simulink library "neuronpoolib"  (Simulink 7.6)
settings: Solver=ode45  StartTime=0.0  StopTime=10.0  RelTol=1e-3
values from neighbouring files (symbols this model uses):
  amp = 1    [excneuroninit.m]
  ampe = 0.5    [excneuroninit.m]
  h = -0.5    [excneuroninit.m]
  maxcon = 10    [excneuroninit.m]
  neurodist = 1    [excneuroninit.m]
  sigslope = 3    [excneuroninit.m]
  tau_u = 0.05    [excneuroninit.m]
  tau_v = 0.1    [excneuroninit.m]
libraries: simulink x20
settings Model: Creator=root  LastModifiedBy=root

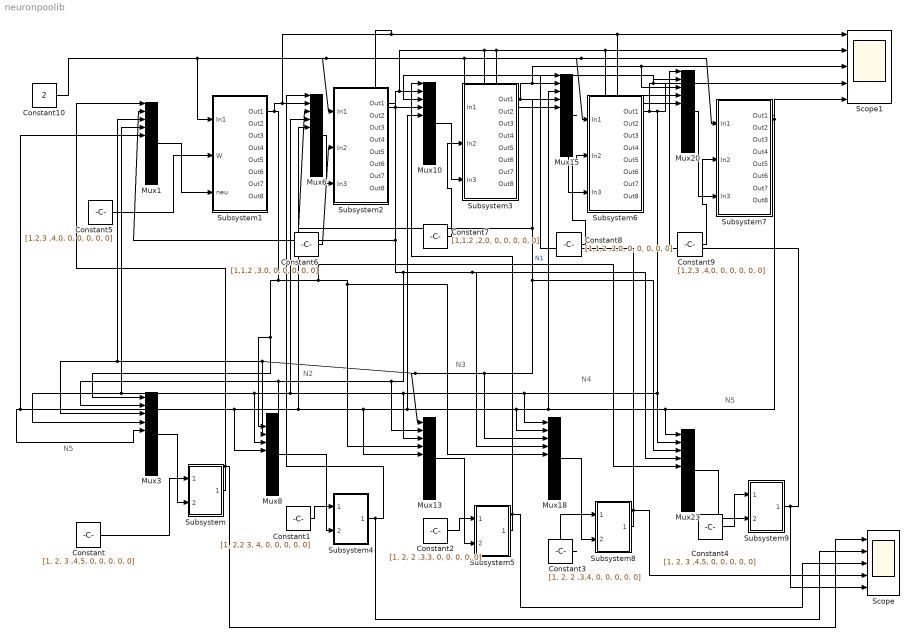
== system neuronpoolib ==
  note: N5
  note: N5
  note: N4
  note: N3
  note: N2
  Constant : Constant  Value=[1, 2, 3 ,4,5, 0, 0, 0, 0, 0]
  Constant1 : Constant  Value=[1, 2,2 3, 4, 0, 0, 0, 0, 0]
  Constant10 : Constant  Value=2
  Constant2 : Constant  Value=[1, 2, 2 ,3,3, 0, 0, 0, 0, 0]
  Constant3 : Constant  Value=[1, 2, 2 ,3,4, 0, 0, 0, 0, 0]
  Constant4 : Constant  Value=[1, 2, 3 ,4,5, 0, 0, 0, 0, 0]
  Constant5 : Constant  Value=[1,2,3 ,4,0, 0, 0, 0, 0, 0]
  Constant6 : Constant  Value=[1,1,2 ,3,0, 0, 0, 0, 0, 0]
  Constant7 : Constant  Value=[1,1,2 ,2,0, 0, 0, 0, 0, 0]
  Constant8 : Constant  Value=[1,1,2 ,3,0, 0, 0, 0, 0, 0]
  Constant9 : Constant  Value=[1,2,3 ,4,0, 0, 0, 0, 0, 0]
  Mux{1,6,10,15,20} (5 alike) : Mux  Inputs=11
  Mux{3,8,13,18,23} (5 alike) : Mux  Inputs=10
  Scope : Scope  NumInputPorts=5
      settings: YMin=-5~-5~-5~-5~-5  YMax=5~5~5~5~5
  Scope1 : Scope  NumInputPorts=5
      settings: YMin=-5~-5~-5~-5~-5  YMax=5~5~5~5~5
  Subsystem : Subsystem
  Subsystem1 : Subsystem
  Subsystem2 : Subsystem
  Subsystem3 : Subsystem
  Subsystem4 : Subsystem
  Subsystem5 : Subsystem
  Subsystem6 : Subsystem
  Subsystem7 : Subsystem
  Subsystem8 : Subsystem
  Subsystem9 : Subsystem
  wires:
  Subsystem1/1(Out1) -> Mux6/2, Mux10/4, Scope1/1, Mux20/5, Mux3/1, Mux8/2, Mux13/4, Mux18/5, Mux23/5  "N1"
  Subsystem2/1(Out1) -> Mux10/2, Mux15/4, Scope1/2, Mux20/4, Mux15/5, Mux3/2, Mux8/1, Mux13/2, Mux18/4, Mux23/4, Mux1/2
  Subsystem3/1(Out1) -> Mux8/3, Mux3/3, Mux1/3, Mux13/1, Mux18/3, Mux23/3, Mux6/3, Mux15/2, Scope1/3, Mux20/3
  Subsystem6/1(Out1) -> Mux18/1, Mux13/3, Mux8/4, Mux3/4, Mux1/4, Mux6/4, Mux23/2, Mux10/3, Mux20/2, Scope1/4
  Subsystem7/1(Out1) -> Mux23/1, Mux18/2, Mux13/5, Mux8/5, Mux3/5, Mux1/5, Mux6/5, Mux10/5, Mux15/3, Scope1/5
  Mux3/1 -> Subsystem/2(port2)
  Mux8/1 -> Subsystem4/2(port2)
  Mux13/1 -> Subsystem5/2(port2)
  Mux18/1 -> Subsystem8/2(port2)
  Mux23/1 -> Subsystem9/2(port2)
  Constant10/1 -> Subsystem2/1(In1), Subsystem7/1(In1), Subsystem6/1(In1), Subsystem3/1(In1), Subsystem1/1(In1)
  Subsystem/1(Out2) -> Mux1/1, Scope/1
  Subsystem4/1(Out2) -> Mux6/1, Scope/2
  Subsystem5/1(Out2) -> Mux10/1, Scope/3
  Subsystem8/1(Out2) -> Mux15/1, Scope/4
  Subsystem9/1(Out2) -> Mux20/1, Scope/5
  Mux1/1 -> Subsystem1/3(neu)
  Mux6/1 -> Subsystem2/3(In3)
  Mux10/1 -> Subsystem3/3(In3)
  Mux15/1 -> Subsystem6/3(In3)
  Mux20/1 -> Subsystem7/3(In3)
  Constant/1 -> Subsystem/1(port1)
  Constant1/1 -> Subsystem4/1(port1)
  ? -> ?
  Constant2/1 -> Subsystem5/1(port1)
  Constant3/1 -> Subsystem8/1(port1)
  Constant4/1 -> Subsystem9/1(port1)
  Constant5/1 -> Subsystem1/2(W)
  Constant6/1 -> Subsystem2/2(In2)
  Constant7/1 -> Subsystem3/2(In2)
  Constant8/1 -> Subsystem6/2(In2)
  Constant9/1 -> Subsystem7/2(In2)

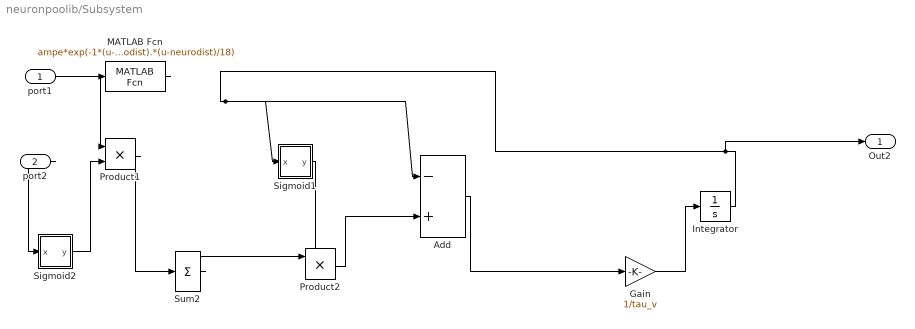
== system neuronpoolib/Subsystem ==
  port1 : Inport
  port2 : Inport  Port=2
  Add : Sum  Inputs=-+
  Gain : Gain  Gain=1/tau_v
  Integrator : Integrator  InitialCondition=1
  MATLAB Fcn : MATLABFcn  MATLABFcn=ampe*exp(-1*(u-neurodist).*(u-neurodist)/18)  OutputDimensions=maxcon
  Product1 : Product  RndMeth=Zero
  Product2 : Product  RndMeth=Zero
  Sigmoid1 : Subsystem  TreatAsAtomicUnit=on  mask{slope=sigslope, offset=0.5}
      mask help: Created by Han, Cheol
      mask Display: plot([10 15 20 25 30 35 40 45 50], [0 0.01 0.1 0.2 0.5 0.8 0.9 0.99 1])
  Sigmoid2 : Subsystem  TreatAsAtomicUnit=on  mask{slope=sigslope, offset=0.5}
      mask help: Created by Han, Cheol
      mask Display: plot([10 15 20 25 30 35 40 45 50], [0 0.01 0.1 0.2 0.5 0.8 0.9 0.99 1])
  Sum2 : Sum  Inputs=+  SaturateOnIntegerOverflow=on
  Out2 : Outport
  wires:
  Add/1 -> Gain/1
  Gain/1 -> Integrator/1
  Integrator/1 -> Add/1, Sigmoid1/1(x), Out2/1
  MATLAB Fcn/1 -> Product1/1
  Sigmoid2/1(y) -> Product1/2
  Product1/1 -> Sum2/1
  Sum2/1 -> Product2/1
  Sigmoid1/1(y) -> Product2/2
  port1/1 -> MATLAB Fcn/1
  port2/1 -> Sigmoid2/1(x)
  Product2/1 -> Add/2

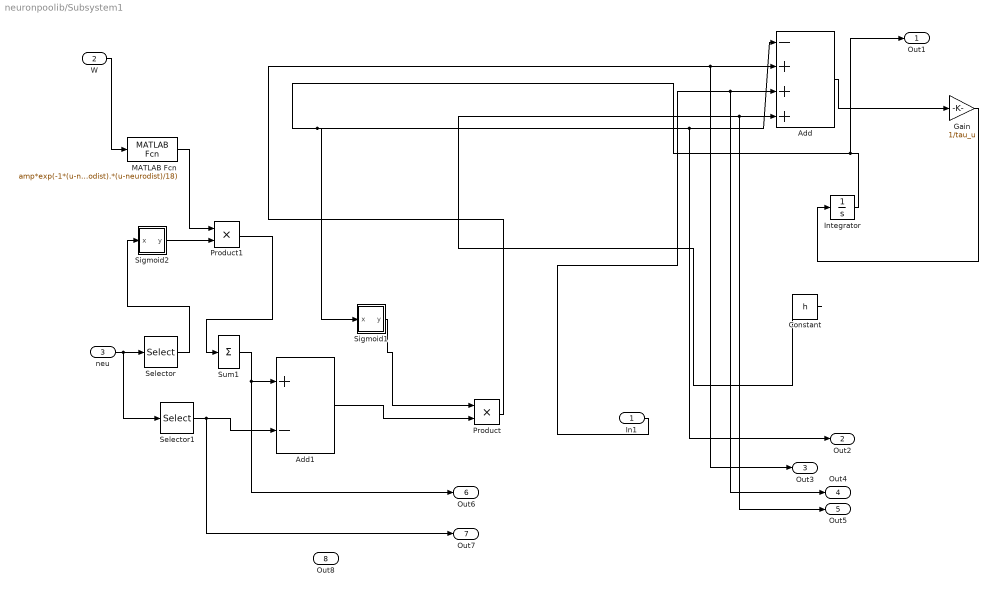
== system neuronpoolib/Subsystem1 ==
  In1 : Inport
  W : Inport  Port=2
  neu : Inport  Port=3
  Add : Sum  Inputs=-+++
  Add1 : Sum  Inputs=+-
  Constant : Constant  Value=h
  Gain : Gain  Gain=1/tau_u
  Integrator : Integrator  InitialCondition=1
  MATLAB Fcn : MATLABFcn  MATLABFcn=amp*exp(-1*(u-neurodist).*(u-neurodist)/18)  OutputDimensions=maxcon
  Product : Product  RndMeth=Zero
  Product1 : Product  RndMeth=Zero
  Selector : Selector  InputPortWidth=maxcon+1  IndexOptions=Starting index (dialog)  Indices=2  OutputSizes=maxcon
  Selector1 : Selector  InputPortWidth=maxcon+1  IndexOptions=Starting index (dialog)  Indices=1  OutputSizes=1
  Sigmoid1 : Subsystem  TreatAsAtomicUnit=on  mask{slope=sigslope, offset=0.5}
      mask help: Created by Han, Cheol
      mask Display: plot([10 15 20 25 30 35 40 45 50], [0 0.01 0.1 0.2 0.5 0.8 0.9 0.99 1])
  Sigmoid2 : Subsystem  TreatAsAtomicUnit=on  mask{slope=sigslope, offset=0.5}
      mask help: Created by Han, Cheol
      mask Display: plot([10 15 20 25 30 35 40 45 50], [0 0.01 0.1 0.2 0.5 0.8 0.9 0.99 1])
  Sum1 : Sum  Inputs=+  SaturateOnIntegerOverflow=on
  Out1 : Outport
  Out2 : Outport  Port=2
  Out3 : Outport  Port=3
  Out4 : Outport  Port=4
  Out5 : Outport  Port=5
  Out6 : Outport  Port=6
  Out7 : Outport  Port=7
  Out8 : Outport  Port=8
  wires:
  Add/1 -> Gain/1
  Gain/1 -> Integrator/1
  Integrator/1 -> Sigmoid1/1(x), Add/1, Out2/1, Out1/1
  Sigmoid1/1(y) -> Product/1
  Product/1 -> Add/2, Out3/1
  In1/1 -> Add/3, Out4/1
  Constant/1 -> Add/4, Out5/1
  neu/1 -> Selector/1, Selector1/1
  Product1/1 -> Sum1/1
  Selector/1 -> Sigmoid2/1(x)
  W/1 -> MATLAB Fcn/1
  MATLAB Fcn/1 -> Product1/1
  Sum1/1 -> Add1/1, Out6/1
  Selector1/1 -> Add1/2, Out7/1
  Sigmoid2/1(y) -> Product1/2
  Add1/1 -> Product/2

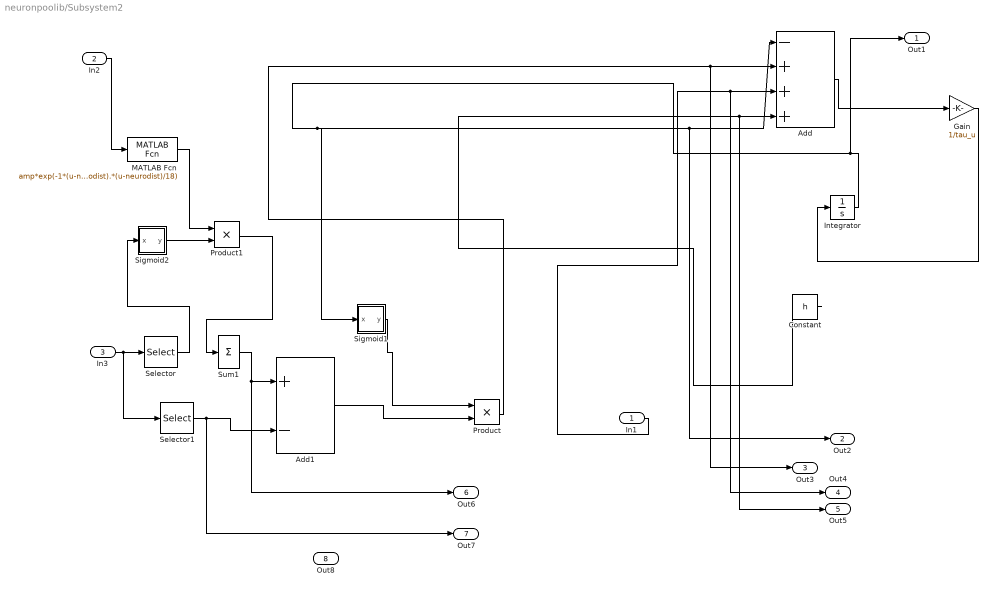
== system neuronpoolib/Subsystem2 ==
  In1 : Inport
  In2 : Inport  Port=2
  In3 : Inport  Port=3
  Add : Sum  Inputs=-+++
  Add1 : Sum  Inputs=+-
  Constant : Constant  Value=h
  Gain : Gain  Gain=1/tau_u
  Integrator : Integrator  InitialCondition=1
  MATLAB Fcn : MATLABFcn  MATLABFcn=amp*exp(-1*(u-neurodist).*(u-neurodist)/18)  OutputDimensions=maxcon
  Product : Product  RndMeth=Zero
  Product1 : Product  RndMeth=Zero
  Selector : Selector  InputPortWidth=maxcon+1  IndexOptions=Starting index (dialog)  Indices=2  OutputSizes=maxcon
  Selector1 : Selector  InputPortWidth=maxcon+1  IndexOptions=Starting index (dialog)  Indices=1  OutputSizes=1
  Sigmoid1 : Subsystem  TreatAsAtomicUnit=on  mask{slope=sigslope, offset=0.5}
      mask help: Created by Han, Cheol
      mask Display: plot([10 15 20 25 30 35 40 45 50], [0 0.01 0.1 0.2 0.5 0.8 0.9 0.99 1])
  Sigmoid2 : Subsystem  TreatAsAtomicUnit=on  mask{slope=sigslope, offset=0.5}
      mask help: Created by Han, Cheol
      mask Display: plot([10 15 20 25 30 35 40 45 50], [0 0.01 0.1 0.2 0.5 0.8 0.9 0.99 1])
  Sum1 : Sum  Inputs=+  SaturateOnIntegerOverflow=on
  Out1 : Outport
  Out2 : Outport  Port=2
  Out3 : Outport  Port=3
  Out4 : Outport  Port=4
  Out5 : Outport  Port=5
  Out6 : Outport  Port=6
  Out7 : Outport  Port=7
  Out8 : Outport  Port=8
  wires:
  Add/1 -> Gain/1
  Gain/1 -> Integrator/1
  Integrator/1 -> Sigmoid1/1(x), Add/1, Out2/1, Out1/1
  Sigmoid1/1(y) -> Product/1
  Product/1 -> Add/2, Out3/1
  In1/1 -> Add/3, Out4/1
  Constant/1 -> Add/4, Out5/1
  In3/1 -> Selector/1, Selector1/1
  Product1/1 -> Sum1/1
  Selector/1 -> Sigmoid2/1(x)
  In2/1 -> MATLAB Fcn/1
  MATLAB Fcn/1 -> Product1/1
  Sum1/1 -> Add1/1, Out6/1
  Selector1/1 -> Add1/2, Out7/1
  Sigmoid2/1(y) -> Product1/2
  Add1/1 -> Product/2

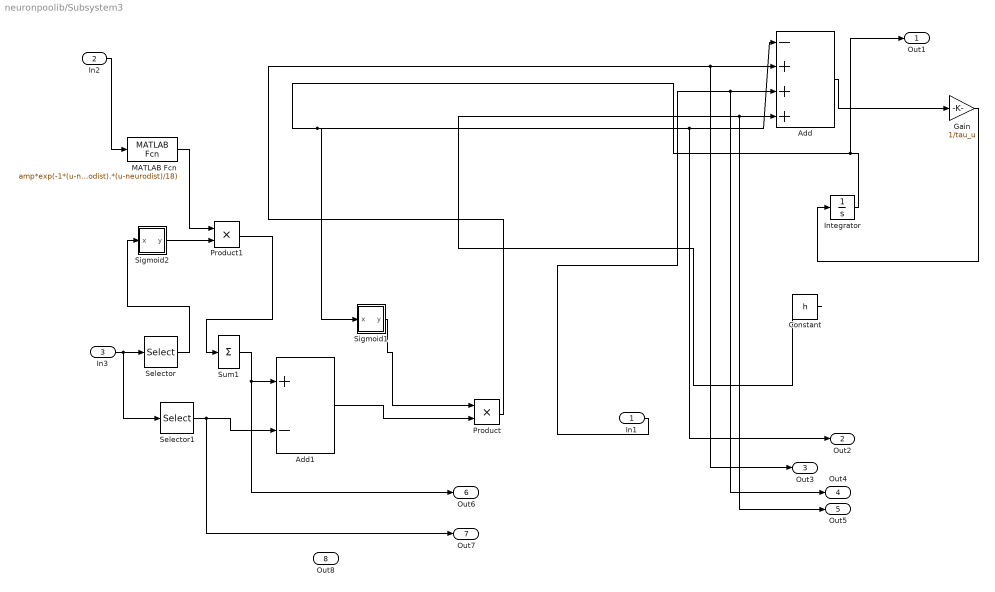
== system neuronpoolib/Subsystem3 ==
  In1 : Inport
  In2 : Inport  Port=2
  In3 : Inport  Port=3
  Add : Sum  Inputs=-+++
  Add1 : Sum  Inputs=+-
  Constant : Constant  Value=h
  Gain : Gain  Gain=1/tau_u
  Integrator : Integrator  InitialCondition=1
  MATLAB Fcn : MATLABFcn  MATLABFcn=amp*exp(-1*(u-neurodist).*(u-neurodist)/18)  OutputDimensions=maxcon
  Product : Product  RndMeth=Zero
  Product1 : Product  RndMeth=Zero
  Selector : Selector  InputPortWidth=maxcon+1  IndexOptions=Starting index (dialog)  Indices=2  OutputSizes=maxcon
  Selector1 : Selector  InputPortWidth=maxcon+1  IndexOptions=Starting index (dialog)  Indices=1  OutputSizes=1
  Sigmoid1 : Subsystem  TreatAsAtomicUnit=on  mask{slope=sigslope, offset=0.5}
      mask help: Created by Han, Cheol
      mask Display: plot([10 15 20 25 30 35 40 45 50], [0 0.01 0.1 0.2 0.5 0.8 0.9 0.99 1])
  Sigmoid2 : Subsystem  TreatAsAtomicUnit=on  mask{slope=sigslope, offset=0.5}
      mask help: Created by Han, Cheol
      mask Display: plot([10 15 20 25 30 35 40 45 50], [0 0.01 0.1 0.2 0.5 0.8 0.9 0.99 1])
  Sum1 : Sum  Inputs=+  SaturateOnIntegerOverflow=on
  Out1 : Outport
  Out2 : Outport  Port=2
  Out3 : Outport  Port=3
  Out4 : Outport  Port=4
  Out5 : Outport  Port=5
  Out6 : Outport  Port=6
  Out7 : Outport  Port=7
  Out8 : Outport  Port=8
  wires:
  Add/1 -> Gain/1
  Gain/1 -> Integrator/1
  Integrator/1 -> Sigmoid1/1(x), Add/1, Out2/1, Out1/1
  Sigmoid1/1(y) -> Product/1
  Product/1 -> Add/2, Out3/1
  In1/1 -> Add/3, Out4/1
  Constant/1 -> Add/4, Out5/1
  In3/1 -> Selector/1, Selector1/1
  Product1/1 -> Sum1/1
  Selector/1 -> Sigmoid2/1(x)
  In2/1 -> MATLAB Fcn/1
  MATLAB Fcn/1 -> Product1/1
  Sum1/1 -> Add1/1, Out6/1
  Selector1/1 -> Add1/2, Out7/1
  Sigmoid2/1(y) -> Product1/2
  Add1/1 -> Product/2

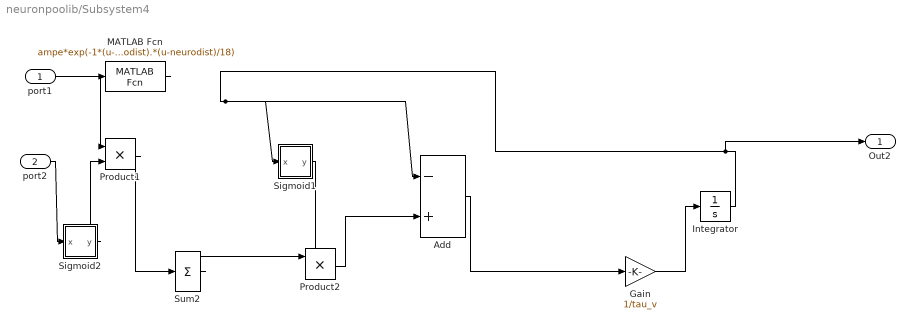
== system neuronpoolib/Subsystem4 ==
  port1 : Inport
  port2 : Inport  Port=2
  Add : Sum  Inputs=-+
  Gain : Gain  Gain=1/tau_v
  Integrator : Integrator  InitialCondition=1
  MATLAB Fcn : MATLABFcn  MATLABFcn=ampe*exp(-1*(u-neurodist).*(u-neurodist)/18)  OutputDimensions=maxcon
  Product1 : Product  RndMeth=Zero
  Product2 : Product  RndMeth=Zero
  Sigmoid1 : Subsystem  TreatAsAtomicUnit=on  mask{slope=sigslope, offset=0.5}
      mask help: Created by Han, Cheol
      mask Display: plot([10 15 20 25 30 35 40 45 50], [0 0.01 0.1 0.2 0.5 0.8 0.9 0.99 1])
  Sigmoid2 : Subsystem  TreatAsAtomicUnit=on  mask{slope=sigslope, offset=0.5}
      mask help: Created by Han, Cheol
      mask Display: plot([10 15 20 25 30 35 40 45 50], [0 0.01 0.1 0.2 0.5 0.8 0.9 0.99 1])
  Sum2 : Sum  Inputs=+  SaturateOnIntegerOverflow=on
  Out2 : Outport
  wires:
  Add/1 -> Gain/1
  Gain/1 -> Integrator/1
  Integrator/1 -> Add/1, Sigmoid1/1(x), Out2/1
  MATLAB Fcn/1 -> Product1/1
  Sigmoid2/1(y) -> Product1/2
  Product1/1 -> Sum2/1
  Sum2/1 -> Product2/1
  Sigmoid1/1(y) -> Product2/2
  port1/1 -> MATLAB Fcn/1
  port2/1 -> Sigmoid2/1(x)
  Product2/1 -> Add/2

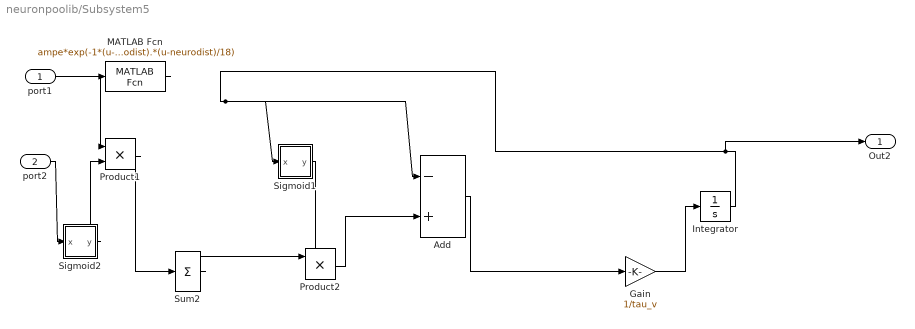
== system neuronpoolib/Subsystem5 ==
  port1 : Inport
  port2 : Inport  Port=2
  Add : Sum  Inputs=-+
  Gain : Gain  Gain=1/tau_v
  Integrator : Integrator  InitialCondition=1
  MATLAB Fcn : MATLABFcn  MATLABFcn=ampe*exp(-1*(u-neurodist).*(u-neurodist)/18)  OutputDimensions=maxcon
  Product1 : Product  RndMeth=Zero
  Product2 : Product  RndMeth=Zero
  Sigmoid1 : Subsystem  TreatAsAtomicUnit=on  mask{slope=sigslope, offset=0.5}
      mask help: Created by Han, Cheol
      mask Display: plot([10 15 20 25 30 35 40 45 50], [0 0.01 0.1 0.2 0.5 0.8 0.9 0.99 1])
  Sigmoid2 : Subsystem  TreatAsAtomicUnit=on  mask{slope=sigslope, offset=0.5}
      mask help: Created by Han, Cheol
      mask Display: plot([10 15 20 25 30 35 40 45 50], [0 0.01 0.1 0.2 0.5 0.8 0.9 0.99 1])
  Sum2 : Sum  Inputs=+  SaturateOnIntegerOverflow=on
  Out2 : Outport
  wires:
  Add/1 -> Gain/1
  Gain/1 -> Integrator/1
  Integrator/1 -> Add/1, Sigmoid1/1(x), Out2/1
  MATLAB Fcn/1 -> Product1/1
  Sigmoid2/1(y) -> Product1/2
  Product1/1 -> Sum2/1
  Sum2/1 -> Product2/1
  Sigmoid1/1(y) -> Product2/2
  port1/1 -> MATLAB Fcn/1
  port2/1 -> Sigmoid2/1(x)
  Product2/1 -> Add/2

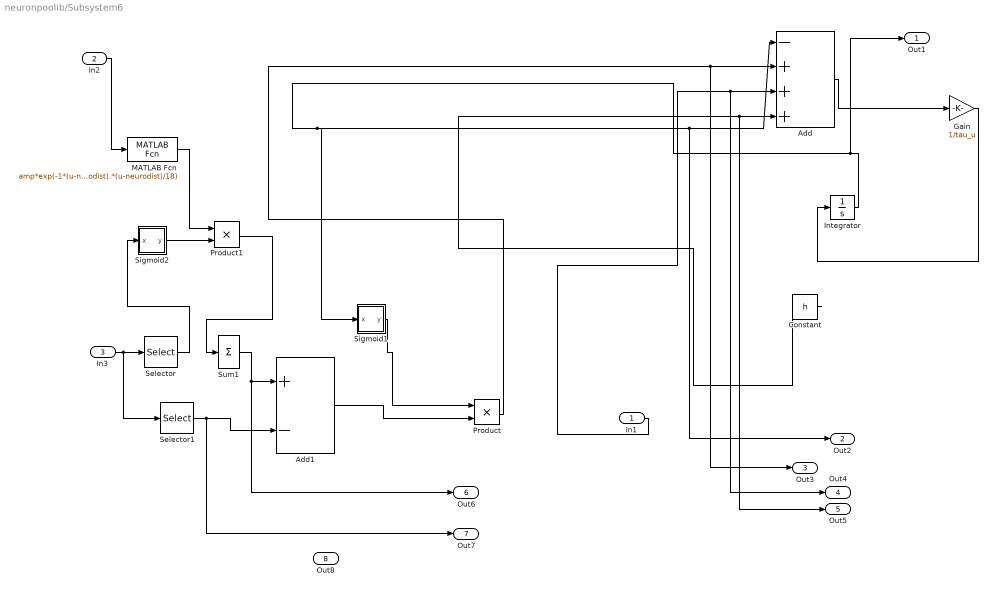
== system neuronpoolib/Subsystem6 ==
  In1 : Inport
  In2 : Inport  Port=2
  In3 : Inport  Port=3
  Add : Sum  Inputs=-+++
  Add1 : Sum  Inputs=+-
  Constant : Constant  Value=h
  Gain : Gain  Gain=1/tau_u
  Integrator : Integrator  InitialCondition=1
  MATLAB Fcn : MATLABFcn  MATLABFcn=amp*exp(-1*(u-neurodist).*(u-neurodist)/18)  OutputDimensions=maxcon
  Product : Product  RndMeth=Zero
  Product1 : Product  RndMeth=Zero
  Selector : Selector  InputPortWidth=maxcon+1  IndexOptions=Starting index (dialog)  Indices=2  OutputSizes=maxcon
  Selector1 : Selector  InputPortWidth=maxcon+1  IndexOptions=Starting index (dialog)  Indices=1  OutputSizes=1
  Sigmoid1 : Subsystem  TreatAsAtomicUnit=on  mask{slope=sigslope, offset=0.5}
      mask help: Created by Han, Cheol
      mask Display: plot([10 15 20 25 30 35 40 45 50], [0 0.01 0.1 0.2 0.5 0.8 0.9 0.99 1])
  Sigmoid2 : Subsystem  TreatAsAtomicUnit=on  mask{slope=sigslope, offset=0.5}
      mask help: Created by Han, Cheol
      mask Display: plot([10 15 20 25 30 35 40 45 50], [0 0.01 0.1 0.2 0.5 0.8 0.9 0.99 1])
  Sum1 : Sum  Inputs=+  SaturateOnIntegerOverflow=on
  Out1 : Outport
  Out2 : Outport  Port=2
  Out3 : Outport  Port=3
  Out4 : Outport  Port=4
  Out5 : Outport  Port=5
  Out6 : Outport  Port=6
  Out7 : Outport  Port=7
  Out8 : Outport  Port=8
  wires:
  Add/1 -> Gain/1
  Gain/1 -> Integrator/1
  Integrator/1 -> Sigmoid1/1(x), Add/1, Out2/1, Out1/1
  Sigmoid1/1(y) -> Product/1
  Product/1 -> Add/2, Out3/1
  In1/1 -> Add/3, Out4/1
  Constant/1 -> Add/4, Out5/1
  In3/1 -> Selector/1, Selector1/1
  Product1/1 -> Sum1/1
  Selector/1 -> Sigmoid2/1(x)
  In2/1 -> MATLAB Fcn/1
  MATLAB Fcn/1 -> Product1/1
  Sum1/1 -> Add1/1, Out6/1
  Selector1/1 -> Add1/2, Out7/1
  Sigmoid2/1(y) -> Product1/2
  Add1/1 -> Product/2

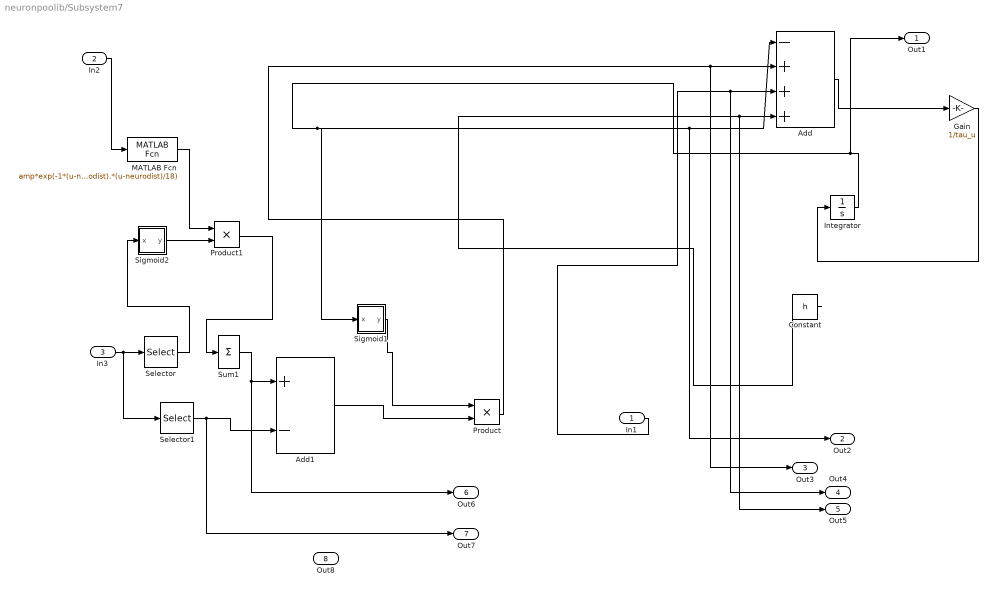
== system neuronpoolib/Subsystem7 ==
  In1 : Inport
  In2 : Inport  Port=2
  In3 : Inport  Port=3
  Add : Sum  Inputs=-+++
  Add1 : Sum  Inputs=+-
  Constant : Constant  Value=h
  Gain : Gain  Gain=1/tau_u
  Integrator : Integrator  InitialCondition=1
  MATLAB Fcn : MATLABFcn  MATLABFcn=amp*exp(-1*(u-neurodist).*(u-neurodist)/18)  OutputDimensions=maxcon
  Product : Product  RndMeth=Zero
  Product1 : Product  RndMeth=Zero
  Selector : Selector  InputPortWidth=maxcon+1  IndexOptions=Starting index (dialog)  Indices=2  OutputSizes=maxcon
  Selector1 : Selector  InputPortWidth=maxcon+1  IndexOptions=Starting index (dialog)  Indices=1  OutputSizes=1
  Sigmoid1 : Subsystem  TreatAsAtomicUnit=on  mask{slope=sigslope, offset=0.5}
      mask help: Created by Han, Cheol
      mask Display: plot([10 15 20 25 30 35 40 45 50], [0 0.01 0.1 0.2 0.5 0.8 0.9 0.99 1])
  Sigmoid2 : Subsystem  TreatAsAtomicUnit=on  mask{slope=sigslope, offset=0.5}
      mask help: Created by Han, Cheol
      mask Display: plot([10 15 20 25 30 35 40 45 50], [0 0.01 0.1 0.2 0.5 0.8 0.9 0.99 1])
  Sum1 : Sum  Inputs=+  SaturateOnIntegerOverflow=on
  Out1 : Outport
  Out2 : Outport  Port=2
  Out3 : Outport  Port=3
  Out4 : Outport  Port=4
  Out5 : Outport  Port=5
  Out6 : Outport  Port=6
  Out7 : Outport  Port=7
  Out8 : Outport  Port=8
  wires:
  Add/1 -> Gain/1
  Gain/1 -> Integrator/1
  Integrator/1 -> Sigmoid1/1(x), Add/1, Out2/1, Out1/1
  Sigmoid1/1(y) -> Product/1
  Product/1 -> Add/2, Out3/1
  In1/1 -> Add/3, Out4/1
  Constant/1 -> Add/4, Out5/1
  In3/1 -> Selector/1, Selector1/1
  Product1/1 -> Sum1/1
  Selector/1 -> Sigmoid2/1(x)
  In2/1 -> MATLAB Fcn/1
  MATLAB Fcn/1 -> Product1/1
  Sum1/1 -> Add1/1, Out6/1
  Selector1/1 -> Add1/2, Out7/1
  Sigmoid2/1(y) -> Product1/2
  Add1/1 -> Product/2

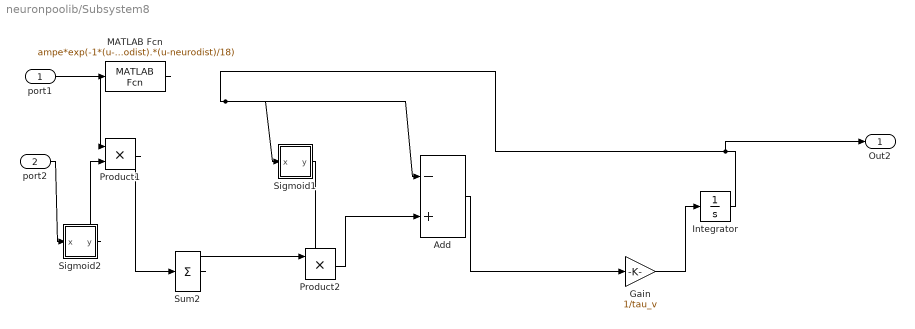
== system neuronpoolib/Subsystem8 ==
  port1 : Inport
  port2 : Inport  Port=2
  Add : Sum  Inputs=-+
  Gain : Gain  Gain=1/tau_v
  Integrator : Integrator  InitialCondition=1
  MATLAB Fcn : MATLABFcn  MATLABFcn=ampe*exp(-1*(u-neurodist).*(u-neurodist)/18)  OutputDimensions=maxcon
  Product1 : Product  RndMeth=Zero
  Product2 : Product  RndMeth=Zero
  Sigmoid1 : Subsystem  TreatAsAtomicUnit=on  mask{slope=sigslope, offset=0.5}
      mask help: Created by Han, Cheol
      mask Display: plot([10 15 20 25 30 35 40 45 50], [0 0.01 0.1 0.2 0.5 0.8 0.9 0.99 1])
  Sigmoid2 : Subsystem  TreatAsAtomicUnit=on  mask{slope=sigslope, offset=0.5}
      mask help: Created by Han, Cheol
      mask Display: plot([10 15 20 25 30 35 40 45 50], [0 0.01 0.1 0.2 0.5 0.8 0.9 0.99 1])
  Sum2 : Sum  Inputs=+  SaturateOnIntegerOverflow=on
  Out2 : Outport
  wires:
  Add/1 -> Gain/1
  Gain/1 -> Integrator/1
  Integrator/1 -> Add/1, Sigmoid1/1(x), Out2/1
  MATLAB Fcn/1 -> Product1/1
  Sigmoid2/1(y) -> Product1/2
  Product1/1 -> Sum2/1
  Sum2/1 -> Product2/1
  Sigmoid1/1(y) -> Product2/2
  port1/1 -> MATLAB Fcn/1
  port2/1 -> Sigmoid2/1(x)
  Product2/1 -> Add/2

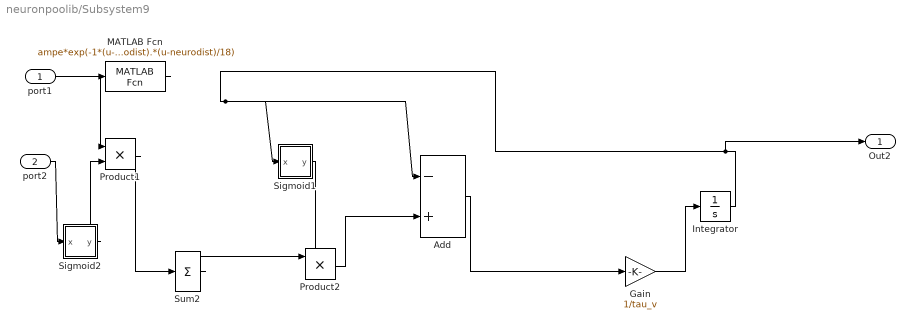
== system neuronpoolib/Subsystem9 ==
  port1 : Inport
  port2 : Inport  Port=2
  Add : Sum  Inputs=-+
  Gain : Gain  Gain=1/tau_v
  Integrator : Integrator  InitialCondition=1
  MATLAB Fcn : MATLABFcn  MATLABFcn=ampe*exp(-1*(u-neurodist).*(u-neurodist)/18)  OutputDimensions=maxcon
  Product1 : Product  RndMeth=Zero
  Product2 : Product  RndMeth=Zero
  Sigmoid1 : Subsystem  TreatAsAtomicUnit=on  mask{slope=sigslope, offset=0.5}
      mask help: Created by Han, Cheol
      mask Display: plot([10 15 20 25 30 35 40 45 50], [0 0.01 0.1 0.2 0.5 0.8 0.9 0.99 1])
  Sigmoid2 : Subsystem  TreatAsAtomicUnit=on  mask{slope=sigslope, offset=0.5}
      mask help: Created by Han, Cheol
      mask Display: plot([10 15 20 25 30 35 40 45 50], [0 0.01 0.1 0.2 0.5 0.8 0.9 0.99 1])
  Sum2 : Sum  Inputs=+  SaturateOnIntegerOverflow=on
  Out2 : Outport
  wires:
  Add/1 -> Gain/1
  Gain/1 -> Integrator/1
  Integrator/1 -> Add/1, Sigmoid1/1(x), Out2/1
  MATLAB Fcn/1 -> Product1/1
  Sigmoid2/1(y) -> Product1/2
  Product1/1 -> Sum2/1
  Sum2/1 -> Product2/1
  Sigmoid1/1(y) -> Product2/2
  port1/1 -> MATLAB Fcn/1
  port2/1 -> Sigmoid2/1(x)
  Product2/1 -> Add/2

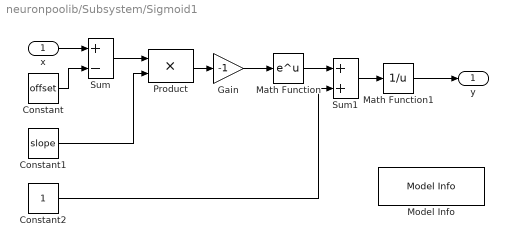
== system neuronpoolib/Subsystem/Sigmoid1 ==
  x : Inport
  Constant : Constant  Value=offset
  Constant1 : Constant  Value=slope
  Constant2 : Constant
  Gain : Gain  Gain=-1  SaturateOnIntegerOverflow=on  OutDataTypeStr=Inherit: Same as input  ParamDataTypeStr=Inherit: Same as input
  Math Function : Math  SaturateOnIntegerOverflow=on
  Math Function1 : Math  Operator=reciprocal  SaturateOnIntegerOverflow=on
  Model Info : simulink/Model-Wide Utilities/Model Info  SystemSampleTime=-1  InitialBlockCM=None  BlockCM=None  Frame=on  DisplayStringWithTags=|  HorizontalTextAlignment=Center  LeftAlignmentValue=0.5  SourceBlockDiagram=untitled  TagMaxNumber=20
      | Model Info
      | %<Creator> Han, Cheol
  Product : Product  SaturateOnIntegerOverflow=on  OutDataTypeStr=Inherit: Same as first input
  Sum : Sum  Inputs=+-  SaturateOnIntegerOverflow=on
  Sum1 : Sum  SaturateOnIntegerOverflow=on
  y : Outport  InitialOutput=0
  wires:
  x/1 -> Sum/1
  Constant/1 -> Sum/2
  Sum/1 -> Product/1
  Constant1/1 -> Product/2
  Product/1 -> Gain/1
  Gain/1 -> Math Function/1
  Math Function/1 -> Sum1/1
  Constant2/1 -> Sum1/2
  Sum1/1 -> Math Function1/1
  Math Function1/1 -> y/1

== system neuronpoolib/Subsystem/Sigmoid2 ==
  x : Inport
  Constant : Constant  Value=offset
  Constant1 : Constant  Value=slope
  Constant2 : Constant
  Gain : Gain  Gain=-1  SaturateOnIntegerOverflow=on  OutDataTypeStr=Inherit: Same as input  ParamDataTypeStr=Inherit: Same as input
  Math Function : Math  SaturateOnIntegerOverflow=on
  Math Function1 : Math  Operator=reciprocal  SaturateOnIntegerOverflow=on
  Model Info : simulink/Model-Wide Utilities/Model Info  SystemSampleTime=-1  InitialBlockCM=None  BlockCM=None  Frame=on  DisplayStringWithTags=|  HorizontalTextAlignment=Center  LeftAlignmentValue=0.5  SourceBlockDiagram=untitled  TagMaxNumber=20
      | Model Info
      | %<Creator> Han, Cheol
  Product : Product  SaturateOnIntegerOverflow=on  OutDataTypeStr=Inherit: Same as first input
  Sum : Sum  Inputs=+-  SaturateOnIntegerOverflow=on
  Sum1 : Sum  SaturateOnIntegerOverflow=on
  y : Outport  InitialOutput=0
  wires:
  x/1 -> Sum/1
  Constant/1 -> Sum/2
  Sum/1 -> Product/1
  Constant1/1 -> Product/2
  Product/1 -> Gain/1
  Gain/1 -> Math Function/1
  Math Function/1 -> Sum1/1
  Constant2/1 -> Sum1/2
  Sum1/1 -> Math Function1/1
  Math Function1/1 -> y/1

== system neuronpoolib/Subsystem1/Sigmoid1 ==
  x : Inport
  Constant : Constant  Value=offset
  Constant1 : Constant  Value=slope
  Constant2 : Constant
  Gain : Gain  Gain=-1  SaturateOnIntegerOverflow=on  OutDataTypeStr=Inherit: Same as input  ParamDataTypeStr=Inherit: Same as input
  Math Function : Math  SaturateOnIntegerOverflow=on
  Math Function1 : Math  Operator=reciprocal  SaturateOnIntegerOverflow=on
  Model Info : simulink/Model-Wide Utilities/Model Info  SystemSampleTime=-1  InitialBlockCM=None  BlockCM=None  Frame=on  DisplayStringWithTags=|  HorizontalTextAlignment=Center  LeftAlignmentValue=0.5  SourceBlockDiagram=untitled  TagMaxNumber=20
      | Model Info
      | %<Creator> Han, Cheol
  Product : Product  SaturateOnIntegerOverflow=on  OutDataTypeStr=Inherit: Same as first input
  Sum : Sum  Inputs=+-  SaturateOnIntegerOverflow=on
  Sum1 : Sum  SaturateOnIntegerOverflow=on
  y : Outport  InitialOutput=0
  wires:
  x/1 -> Sum/1
  Constant/1 -> Sum/2
  Sum/1 -> Product/1
  Constant1/1 -> Product/2
  Product/1 -> Gain/1
  Gain/1 -> Math Function/1
  Math Function/1 -> Sum1/1
  Constant2/1 -> Sum1/2
  Sum1/1 -> Math Function1/1
  Math Function1/1 -> y/1

== system neuronpoolib/Subsystem1/Sigmoid2 ==
  x : Inport
  Constant : Constant  Value=offset
  Constant1 : Constant  Value=slope
  Constant2 : Constant
  Gain : Gain  Gain=-1  SaturateOnIntegerOverflow=on  OutDataTypeStr=Inherit: Same as input  ParamDataTypeStr=Inherit: Same as input
  Math Function : Math  SaturateOnIntegerOverflow=on
  Math Function1 : Math  Operator=reciprocal  SaturateOnIntegerOverflow=on
  Model Info : simulink/Model-Wide Utilities/Model Info  SystemSampleTime=-1  InitialBlockCM=None  BlockCM=None  Frame=on  DisplayStringWithTags=|  HorizontalTextAlignment=Center  LeftAlignmentValue=0.5  SourceBlockDiagram=untitled  TagMaxNumber=20
      | Model Info
      | %<Creator> Han, Cheol
  Product : Product  SaturateOnIntegerOverflow=on  OutDataTypeStr=Inherit: Same as first input
  Sum : Sum  Inputs=+-  SaturateOnIntegerOverflow=on
  Sum1 : Sum  SaturateOnIntegerOverflow=on
  y : Outport  InitialOutput=0
  wires:
  x/1 -> Sum/1
  Constant/1 -> Sum/2
  Sum/1 -> Product/1
  Constant1/1 -> Product/2
  Product/1 -> Gain/1
  Gain/1 -> Math Function/1
  Math Function/1 -> Sum1/1
  Constant2/1 -> Sum1/2
  Sum1/1 -> Math Function1/1
  Math Function1/1 -> y/1

== system neuronpoolib/Subsystem2/Sigmoid1 ==
  x : Inport
  Constant : Constant  Value=offset
  Constant1 : Constant  Value=slope
  Constant2 : Constant
  Gain : Gain  Gain=-1  SaturateOnIntegerOverflow=on  OutDataTypeStr=Inherit: Same as input  ParamDataTypeStr=Inherit: Same as input
  Math Function : Math  SaturateOnIntegerOverflow=on
  Math Function1 : Math  Operator=reciprocal  SaturateOnIntegerOverflow=on
  Model Info : simulink/Model-Wide Utilities/Model Info  SystemSampleTime=-1  InitialBlockCM=None  BlockCM=None  Frame=on  DisplayStringWithTags=|  HorizontalTextAlignment=Center  LeftAlignmentValue=0.5  SourceBlockDiagram=untitled  TagMaxNumber=20
      | Model Info
      | %<Creator> Han, Cheol
  Product : Product  SaturateOnIntegerOverflow=on  OutDataTypeStr=Inherit: Same as first input
  Sum : Sum  Inputs=+-  SaturateOnIntegerOverflow=on
  Sum1 : Sum  SaturateOnIntegerOverflow=on
  y : Outport  InitialOutput=0
  wires:
  x/1 -> Sum/1
  Constant/1 -> Sum/2
  Sum/1 -> Product/1
  Constant1/1 -> Product/2
  Product/1 -> Gain/1
  Gain/1 -> Math Function/1
  Math Function/1 -> Sum1/1
  Constant2/1 -> Sum1/2
  Sum1/1 -> Math Function1/1
  Math Function1/1 -> y/1

== system neuronpoolib/Subsystem2/Sigmoid2 ==
  x : Inport
  Constant : Constant  Value=offset
  Constant1 : Constant  Value=slope
  Constant2 : Constant
  Gain : Gain  Gain=-1  SaturateOnIntegerOverflow=on  OutDataTypeStr=Inherit: Same as input  ParamDataTypeStr=Inherit: Same as input
  Math Function : Math  SaturateOnIntegerOverflow=on
  Math Function1 : Math  Operator=reciprocal  SaturateOnIntegerOverflow=on
  Model Info : simulink/Model-Wide Utilities/Model Info  SystemSampleTime=-1  InitialBlockCM=None  BlockCM=None  Frame=on  DisplayStringWithTags=|  HorizontalTextAlignment=Center  LeftAlignmentValue=0.5  SourceBlockDiagram=untitled  TagMaxNumber=20
      | Model Info
      | %<Creator> Han, Cheol
  Product : Product  SaturateOnIntegerOverflow=on  OutDataTypeStr=Inherit: Same as first input
  Sum : Sum  Inputs=+-  SaturateOnIntegerOverflow=on
  Sum1 : Sum  SaturateOnIntegerOverflow=on
  y : Outport  InitialOutput=0
  wires:
  x/1 -> Sum/1
  Constant/1 -> Sum/2
  Sum/1 -> Product/1
  Constant1/1 -> Product/2
  Product/1 -> Gain/1
  Gain/1 -> Math Function/1
  Math Function/1 -> Sum1/1
  Constant2/1 -> Sum1/2
  Sum1/1 -> Math Function1/1
  Math Function1/1 -> y/1

== system neuronpoolib/Subsystem3/Sigmoid1 ==
  x : Inport
  Constant : Constant  Value=offset
  Constant1 : Constant  Value=slope
  Constant2 : Constant
  Gain : Gain  Gain=-1  SaturateOnIntegerOverflow=on  OutDataTypeStr=Inherit: Same as input  ParamDataTypeStr=Inherit: Same as input
  Math Function : Math  SaturateOnIntegerOverflow=on
  Math Function1 : Math  Operator=reciprocal  SaturateOnIntegerOverflow=on
  Model Info : simulink/Model-Wide Utilities/Model Info  SystemSampleTime=-1  InitialBlockCM=None  BlockCM=None  Frame=on  DisplayStringWithTags=|  HorizontalTextAlignment=Center  LeftAlignmentValue=0.5  SourceBlockDiagram=untitled  TagMaxNumber=20
      | Model Info
      | %<Creator> Han, Cheol
  Product : Product  SaturateOnIntegerOverflow=on  OutDataTypeStr=Inherit: Same as first input
  Sum : Sum  Inputs=+-  SaturateOnIntegerOverflow=on
  Sum1 : Sum  SaturateOnIntegerOverflow=on
  y : Outport  InitialOutput=0
  wires:
  x/1 -> Sum/1
  Constant/1 -> Sum/2
  Sum/1 -> Product/1
  Constant1/1 -> Product/2
  Product/1 -> Gain/1
  Gain/1 -> Math Function/1
  Math Function/1 -> Sum1/1
  Constant2/1 -> Sum1/2
  Sum1/1 -> Math Function1/1
  Math Function1/1 -> y/1

== system neuronpoolib/Subsystem3/Sigmoid2 ==
  x : Inport
  Constant : Constant  Value=offset
  Constant1 : Constant  Value=slope
  Constant2 : Constant
  Gain : Gain  Gain=-1  SaturateOnIntegerOverflow=on  OutDataTypeStr=Inherit: Same as input  ParamDataTypeStr=Inherit: Same as input
  Math Function : Math  SaturateOnIntegerOverflow=on
  Math Function1 : Math  Operator=reciprocal  SaturateOnIntegerOverflow=on
  Model Info : simulink/Model-Wide Utilities/Model Info  SystemSampleTime=-1  InitialBlockCM=None  BlockCM=None  Frame=on  DisplayStringWithTags=|  HorizontalTextAlignment=Center  LeftAlignmentValue=0.5  SourceBlockDiagram=untitled  TagMaxNumber=20
      | Model Info
      | %<Creator> Han, Cheol
  Product : Product  SaturateOnIntegerOverflow=on  OutDataTypeStr=Inherit: Same as first input
  Sum : Sum  Inputs=+-  SaturateOnIntegerOverflow=on
  Sum1 : Sum  SaturateOnIntegerOverflow=on
  y : Outport  InitialOutput=0
  wires:
  x/1 -> Sum/1
  Constant/1 -> Sum/2
  Sum/1 -> Product/1
  Constant1/1 -> Product/2
  Product/1 -> Gain/1
  Gain/1 -> Math Function/1
  Math Function/1 -> Sum1/1
  Constant2/1 -> Sum1/2
  Sum1/1 -> Math Function1/1
  Math Function1/1 -> y/1

== system neuronpoolib/Subsystem4/Sigmoid1 ==
  x : Inport
  Constant : Constant  Value=offset
  Constant1 : Constant  Value=slope
  Constant2 : Constant
  Gain : Gain  Gain=-1  SaturateOnIntegerOverflow=on  OutDataTypeStr=Inherit: Same as input  ParamDataTypeStr=Inherit: Same as input
  Math Function : Math  SaturateOnIntegerOverflow=on
  Math Function1 : Math  Operator=reciprocal  SaturateOnIntegerOverflow=on
  Model Info : simulink/Model-Wide Utilities/Model Info  SystemSampleTime=-1  InitialBlockCM=None  BlockCM=None  Frame=on  DisplayStringWithTags=|  HorizontalTextAlignment=Center  LeftAlignmentValue=0.5  SourceBlockDiagram=untitled  TagMaxNumber=20
      | Model Info
      | %<Creator> Han, Cheol
  Product : Product  SaturateOnIntegerOverflow=on  OutDataTypeStr=Inherit: Same as first input
  Sum : Sum  Inputs=+-  SaturateOnIntegerOverflow=on
  Sum1 : Sum  SaturateOnIntegerOverflow=on
  y : Outport  InitialOutput=0
  wires:
  x/1 -> Sum/1
  Constant/1 -> Sum/2
  Sum/1 -> Product/1
  Constant1/1 -> Product/2
  Product/1 -> Gain/1
  Gain/1 -> Math Function/1
  Math Function/1 -> Sum1/1
  Constant2/1 -> Sum1/2
  Sum1/1 -> Math Function1/1
  Math Function1/1 -> y/1

== system neuronpoolib/Subsystem4/Sigmoid2 ==
  x : Inport
  Constant : Constant  Value=offset
  Constant1 : Constant  Value=slope
  Constant2 : Constant
  Gain : Gain  Gain=-1  SaturateOnIntegerOverflow=on  OutDataTypeStr=Inherit: Same as input  ParamDataTypeStr=Inherit: Same as input
  Math Function : Math  SaturateOnIntegerOverflow=on
  Math Function1 : Math  Operator=reciprocal  SaturateOnIntegerOverflow=on
  Model Info : simulink/Model-Wide Utilities/Model Info  SystemSampleTime=-1  InitialBlockCM=None  BlockCM=None  Frame=on  DisplayStringWithTags=|  HorizontalTextAlignment=Center  LeftAlignmentValue=0.5  SourceBlockDiagram=untitled  TagMaxNumber=20
      | Model Info
      | %<Creator> Han, Cheol
  Product : Product  SaturateOnIntegerOverflow=on  OutDataTypeStr=Inherit: Same as first input
  Sum : Sum  Inputs=+-  SaturateOnIntegerOverflow=on
  Sum1 : Sum  SaturateOnIntegerOverflow=on
  y : Outport  InitialOutput=0
  wires:
  x/1 -> Sum/1
  Constant/1 -> Sum/2
  Sum/1 -> Product/1
  Constant1/1 -> Product/2
  Product/1 -> Gain/1
  Gain/1 -> Math Function/1
  Math Function/1 -> Sum1/1
  Constant2/1 -> Sum1/2
  Sum1/1 -> Math Function1/1
  Math Function1/1 -> y/1

== system neuronpoolib/Subsystem5/Sigmoid1 ==
  x : Inport
  Constant : Constant  Value=offset
  Constant1 : Constant  Value=slope
  Constant2 : Constant
  Gain : Gain  Gain=-1  SaturateOnIntegerOverflow=on  OutDataTypeStr=Inherit: Same as input  ParamDataTypeStr=Inherit: Same as input
  Math Function : Math  SaturateOnIntegerOverflow=on
  Math Function1 : Math  Operator=reciprocal  SaturateOnIntegerOverflow=on
  Model Info : simulink/Model-Wide Utilities/Model Info  SystemSampleTime=-1  InitialBlockCM=None  BlockCM=None  Frame=on  DisplayStringWithTags=|  HorizontalTextAlignment=Center  LeftAlignmentValue=0.5  SourceBlockDiagram=untitled  TagMaxNumber=20
      | Model Info
      | %<Creator> Han, Cheol
  Product : Product  SaturateOnIntegerOverflow=on  OutDataTypeStr=Inherit: Same as first input
  Sum : Sum  Inputs=+-  SaturateOnIntegerOverflow=on
  Sum1 : Sum  SaturateOnIntegerOverflow=on
  y : Outport  InitialOutput=0
  wires:
  x/1 -> Sum/1
  Constant/1 -> Sum/2
  Sum/1 -> Product/1
  Constant1/1 -> Product/2
  Product/1 -> Gain/1
  Gain/1 -> Math Function/1
  Math Function/1 -> Sum1/1
  Constant2/1 -> Sum1/2
  Sum1/1 -> Math Function1/1
  Math Function1/1 -> y/1

== system neuronpoolib/Subsystem5/Sigmoid2 ==
  x : Inport
  Constant : Constant  Value=offset
  Constant1 : Constant  Value=slope
  Constant2 : Constant
  Gain : Gain  Gain=-1  SaturateOnIntegerOverflow=on  OutDataTypeStr=Inherit: Same as input  ParamDataTypeStr=Inherit: Same as input
  Math Function : Math  SaturateOnIntegerOverflow=on
  Math Function1 : Math  Operator=reciprocal  SaturateOnIntegerOverflow=on
  Model Info : simulink/Model-Wide Utilities/Model Info  SystemSampleTime=-1  InitialBlockCM=None  BlockCM=None  Frame=on  DisplayStringWithTags=|  HorizontalTextAlignment=Center  LeftAlignmentValue=0.5  SourceBlockDiagram=untitled  TagMaxNumber=20
      | Model Info
      | %<Creator> Han, Cheol
  Product : Product  SaturateOnIntegerOverflow=on  OutDataTypeStr=Inherit: Same as first input
  Sum : Sum  Inputs=+-  SaturateOnIntegerOverflow=on
  Sum1 : Sum  SaturateOnIntegerOverflow=on
  y : Outport  InitialOutput=0
  wires:
  x/1 -> Sum/1
  Constant/1 -> Sum/2
  Sum/1 -> Product/1
  Constant1/1 -> Product/2
  Product/1 -> Gain/1
  Gain/1 -> Math Function/1
  Math Function/1 -> Sum1/1
  Constant2/1 -> Sum1/2
  Sum1/1 -> Math Function1/1
  Math Function1/1 -> y/1

== system neuronpoolib/Subsystem6/Sigmoid1 ==
  x : Inport
  Constant : Constant  Value=offset
  Constant1 : Constant  Value=slope
  Constant2 : Constant
  Gain : Gain  Gain=-1  SaturateOnIntegerOverflow=on  OutDataTypeStr=Inherit: Same as input  ParamDataTypeStr=Inherit: Same as input
  Math Function : Math  SaturateOnIntegerOverflow=on
  Math Function1 : Math  Operator=reciprocal  SaturateOnIntegerOverflow=on
  Model Info : simulink/Model-Wide Utilities/Model Info  SystemSampleTime=-1  InitialBlockCM=None  BlockCM=None  Frame=on  DisplayStringWithTags=|  HorizontalTextAlignment=Center  LeftAlignmentValue=0.5  SourceBlockDiagram=untitled  TagMaxNumber=20
      | Model Info
      | %<Creator> Han, Cheol
  Product : Product  SaturateOnIntegerOverflow=on  OutDataTypeStr=Inherit: Same as first input
  Sum : Sum  Inputs=+-  SaturateOnIntegerOverflow=on
  Sum1 : Sum  SaturateOnIntegerOverflow=on
  y : Outport  InitialOutput=0
  wires:
  x/1 -> Sum/1
  Constant/1 -> Sum/2
  Sum/1 -> Product/1
  Constant1/1 -> Product/2
  Product/1 -> Gain/1
  Gain/1 -> Math Function/1
  Math Function/1 -> Sum1/1
  Constant2/1 -> Sum1/2
  Sum1/1 -> Math Function1/1
  Math Function1/1 -> y/1

== system neuronpoolib/Subsystem6/Sigmoid2 ==
  x : Inport
  Constant : Constant  Value=offset
  Constant1 : Constant  Value=slope
  Constant2 : Constant
  Gain : Gain  Gain=-1  SaturateOnIntegerOverflow=on  OutDataTypeStr=Inherit: Same as input  ParamDataTypeStr=Inherit: Same as input
  Math Function : Math  SaturateOnIntegerOverflow=on
  Math Function1 : Math  Operator=reciprocal  SaturateOnIntegerOverflow=on
  Model Info : simulink/Model-Wide Utilities/Model Info  SystemSampleTime=-1  InitialBlockCM=None  BlockCM=None  Frame=on  DisplayStringWithTags=|  HorizontalTextAlignment=Center  LeftAlignmentValue=0.5  SourceBlockDiagram=untitled  TagMaxNumber=20
      | Model Info
      | %<Creator> Han, Cheol
  Product : Product  SaturateOnIntegerOverflow=on  OutDataTypeStr=Inherit: Same as first input
  Sum : Sum  Inputs=+-  SaturateOnIntegerOverflow=on
  Sum1 : Sum  SaturateOnIntegerOverflow=on
  y : Outport  InitialOutput=0
  wires:
  x/1 -> Sum/1
  Constant/1 -> Sum/2
  Sum/1 -> Product/1
  Constant1/1 -> Product/2
  Product/1 -> Gain/1
  Gain/1 -> Math Function/1
  Math Function/1 -> Sum1/1
  Constant2/1 -> Sum1/2
  Sum1/1 -> Math Function1/1
  Math Function1/1 -> y/1

== system neuronpoolib/Subsystem7/Sigmoid1 ==
  x : Inport
  Constant : Constant  Value=offset
  Constant1 : Constant  Value=slope
  Constant2 : Constant
  Gain : Gain  Gain=-1  SaturateOnIntegerOverflow=on  OutDataTypeStr=Inherit: Same as input  ParamDataTypeStr=Inherit: Same as input
  Math Function : Math  SaturateOnIntegerOverflow=on
  Math Function1 : Math  Operator=reciprocal  SaturateOnIntegerOverflow=on
  Model Info : simulink/Model-Wide Utilities/Model Info  SystemSampleTime=-1  InitialBlockCM=None  BlockCM=None  Frame=on  DisplayStringWithTags=|  HorizontalTextAlignment=Center  LeftAlignmentValue=0.5  SourceBlockDiagram=untitled  TagMaxNumber=20
      | Model Info
      | %<Creator> Han, Cheol
  Product : Product  SaturateOnIntegerOverflow=on  OutDataTypeStr=Inherit: Same as first input
  Sum : Sum  Inputs=+-  SaturateOnIntegerOverflow=on
  Sum1 : Sum  SaturateOnIntegerOverflow=on
  y : Outport  InitialOutput=0
  wires:
  x/1 -> Sum/1
  Constant/1 -> Sum/2
  Sum/1 -> Product/1
  Constant1/1 -> Product/2
  Product/1 -> Gain/1
  Gain/1 -> Math Function/1
  Math Function/1 -> Sum1/1
  Constant2/1 -> Sum1/2
  Sum1/1 -> Math Function1/1
  Math Function1/1 -> y/1

== system neuronpoolib/Subsystem7/Sigmoid2 ==
  x : Inport
  Constant : Constant  Value=offset
  Constant1 : Constant  Value=slope
  Constant2 : Constant
  Gain : Gain  Gain=-1  SaturateOnIntegerOverflow=on  OutDataTypeStr=Inherit: Same as input  ParamDataTypeStr=Inherit: Same as input
  Math Function : Math  SaturateOnIntegerOverflow=on
  Math Function1 : Math  Operator=reciprocal  SaturateOnIntegerOverflow=on
  Model Info : simulink/Model-Wide Utilities/Model Info  SystemSampleTime=-1  InitialBlockCM=None  BlockCM=None  Frame=on  DisplayStringWithTags=|  HorizontalTextAlignment=Center  LeftAlignmentValue=0.5  SourceBlockDiagram=untitled  TagMaxNumber=20
      | Model Info
      | %<Creator> Han, Cheol
  Product : Product  SaturateOnIntegerOverflow=on  OutDataTypeStr=Inherit: Same as first input
  Sum : Sum  Inputs=+-  SaturateOnIntegerOverflow=on
  Sum1 : Sum  SaturateOnIntegerOverflow=on
  y : Outport  InitialOutput=0
  wires:
  x/1 -> Sum/1
  Constant/1 -> Sum/2
  Sum/1 -> Product/1
  Constant1/1 -> Product/2
  Product/1 -> Gain/1
  Gain/1 -> Math Function/1
  Math Function/1 -> Sum1/1
  Constant2/1 -> Sum1/2
  Sum1/1 -> Math Function1/1
  Math Function1/1 -> y/1

== system neuronpoolib/Subsystem8/Sigmoid1 ==
  x : Inport
  Constant : Constant  Value=offset
  Constant1 : Constant  Value=slope
  Constant2 : Constant
  Gain : Gain  Gain=-1  SaturateOnIntegerOverflow=on  OutDataTypeStr=Inherit: Same as input  ParamDataTypeStr=Inherit: Same as input
  Math Function : Math  SaturateOnIntegerOverflow=on
  Math Function1 : Math  Operator=reciprocal  SaturateOnIntegerOverflow=on
  Model Info : simulink/Model-Wide Utilities/Model Info  SystemSampleTime=-1  InitialBlockCM=None  BlockCM=None  Frame=on  DisplayStringWithTags=|  HorizontalTextAlignment=Center  LeftAlignmentValue=0.5  SourceBlockDiagram=untitled  TagMaxNumber=20
      | Model Info
      | %<Creator> Han, Cheol
  Product : Product  SaturateOnIntegerOverflow=on  OutDataTypeStr=Inherit: Same as first input
  Sum : Sum  Inputs=+-  SaturateOnIntegerOverflow=on
  Sum1 : Sum  SaturateOnIntegerOverflow=on
  y : Outport  InitialOutput=0
  wires:
  x/1 -> Sum/1
  Constant/1 -> Sum/2
  Sum/1 -> Product/1
  Constant1/1 -> Product/2
  Product/1 -> Gain/1
  Gain/1 -> Math Function/1
  Math Function/1 -> Sum1/1
  Constant2/1 -> Sum1/2
  Sum1/1 -> Math Function1/1
  Math Function1/1 -> y/1

== system neuronpoolib/Subsystem8/Sigmoid2 ==
  x : Inport
  Constant : Constant  Value=offset
  Constant1 : Constant  Value=slope
  Constant2 : Constant
  Gain : Gain  Gain=-1  SaturateOnIntegerOverflow=on  OutDataTypeStr=Inherit: Same as input  ParamDataTypeStr=Inherit: Same as input
  Math Function : Math  SaturateOnIntegerOverflow=on
  Math Function1 : Math  Operator=reciprocal  SaturateOnIntegerOverflow=on
  Model Info : simulink/Model-Wide Utilities/Model Info  SystemSampleTime=-1  InitialBlockCM=None  BlockCM=None  Frame=on  DisplayStringWithTags=|  HorizontalTextAlignment=Center  LeftAlignmentValue=0.5  SourceBlockDiagram=untitled  TagMaxNumber=20
      | Model Info
      | %<Creator> Han, Cheol
  Product : Product  SaturateOnIntegerOverflow=on  OutDataTypeStr=Inherit: Same as first input
  Sum : Sum  Inputs=+-  SaturateOnIntegerOverflow=on
  Sum1 : Sum  SaturateOnIntegerOverflow=on
  y : Outport  InitialOutput=0
  wires:
  x/1 -> Sum/1
  Constant/1 -> Sum/2
  Sum/1 -> Product/1
  Constant1/1 -> Product/2
  Product/1 -> Gain/1
  Gain/1 -> Math Function/1
  Math Function/1 -> Sum1/1
  Constant2/1 -> Sum1/2
  Sum1/1 -> Math Function1/1
  Math Function1/1 -> y/1

== system neuronpoolib/Subsystem9/Sigmoid1 ==
  x : Inport
  Constant : Constant  Value=offset
  Constant1 : Constant  Value=slope
  Constant2 : Constant
  Gain : Gain  Gain=-1  SaturateOnIntegerOverflow=on  OutDataTypeStr=Inherit: Same as input  ParamDataTypeStr=Inherit: Same as input
  Math Function : Math  SaturateOnIntegerOverflow=on
  Math Function1 : Math  Operator=reciprocal  SaturateOnIntegerOverflow=on
  Model Info : simulink/Model-Wide Utilities/Model Info  SystemSampleTime=-1  InitialBlockCM=None  BlockCM=None  Frame=on  DisplayStringWithTags=|  HorizontalTextAlignment=Center  LeftAlignmentValue=0.5  SourceBlockDiagram=untitled  TagMaxNumber=20
      | Model Info
      | %<Creator> Han, Cheol
  Product : Product  SaturateOnIntegerOverflow=on  OutDataTypeStr=Inherit: Same as first input
  Sum : Sum  Inputs=+-  SaturateOnIntegerOverflow=on
  Sum1 : Sum  SaturateOnIntegerOverflow=on
  y : Outport  InitialOutput=0
  wires:
  x/1 -> Sum/1
  Constant/1 -> Sum/2
  Sum/1 -> Product/1
  Constant1/1 -> Product/2
  Product/1 -> Gain/1
  Gain/1 -> Math Function/1
  Math Function/1 -> Sum1/1
  Constant2/1 -> Sum1/2
  Sum1/1 -> Math Function1/1
  Math Function1/1 -> y/1

== system neuronpoolib/Subsystem9/Sigmoid2 ==
  x : Inport
  Constant : Constant  Value=offset
  Constant1 : Constant  Value=slope
  Constant2 : Constant
  Gain : Gain  Gain=-1  SaturateOnIntegerOverflow=on  OutDataTypeStr=Inherit: Same as input  ParamDataTypeStr=Inherit: Same as input
  Math Function : Math  SaturateOnIntegerOverflow=on
  Math Function1 : Math  Operator=reciprocal  SaturateOnIntegerOverflow=on
  Model Info : simulink/Model-Wide Utilities/Model Info  SystemSampleTime=-1  InitialBlockCM=None  BlockCM=None  Frame=on  DisplayStringWithTags=|  HorizontalTextAlignment=Center  LeftAlignmentValue=0.5  SourceBlockDiagram=untitled  TagMaxNumber=20
      | Model Info
      | %<Creator> Han, Cheol
  Product : Product  SaturateOnIntegerOverflow=on  OutDataTypeStr=Inherit: Same as first input
  Sum : Sum  Inputs=+-  SaturateOnIntegerOverflow=on
  Sum1 : Sum  SaturateOnIntegerOverflow=on
  y : Outport  InitialOutput=0
  wires:
  x/1 -> Sum/1
  Constant/1 -> Sum/2
  Sum/1 -> Product/1
  Constant1/1 -> Product/2
  Product/1 -> Gain/1
  Gain/1 -> Math Function/1
  Math Function/1 -> Sum1/1
  Constant2/1 -> Sum1/2
  Sum1/1 -> Math Function1/1
  Math Function1/1 -> y/1
